simulink model "cube_2d_simulation_model_mpc"  (R2016b)
settings: Solver=VariableStepAuto  StartTime=0.0  StopTime=6  FixedStep=0.001  RelTol=1e-3  EnableMultiTasking=on
PreLoadFcn:
  | cubeinit
InitFcn:
  | cubeparameters
values from neighbouring files (symbols this model uses):
  g = 9.81    [MPC_Parameters.m]
  x0 = [deg2rad(2) 0]'    [MPC_init.m]    (also in MPC_simulation_linearized_system.m; MPC_simulation_nonlinearized_system.m; fastMPC.m)
undefined symbols (not defined in the file or in its folder): a_max, a_scaling, cube, deg_, imu_intended_alignment, imu_misalignment, motor, r_cube2imu, sensor_seed, T_onboard, Ts, w_max, w_scaling, wheel
libraries: cube_lib x9, simulink x6, cubex_simulation x3, stm32f4_io_lib x2
settings Model: Creator=Stefan  LastModifiedBy=Wall
settings DataIOCC: LimitDataPoints=on
settings OptimizationCC: LifeSpan=inf
settings DebuggingCC: AlgebraicLoopMsg=none  AllowSymbolicDim=off  SFUnexpectedBacktrackingDiag=warning  SFNoUnconditionalDefaultTransitionDiag=warning  SFExecutionAtInitializationDiag=none
settings ModelReferenceCC: PropagateSignalLabelsOutOfModel=off
settings GRTTargetCC: TargetLangStandard=C89/C90 (ANSI)
settings ConfigComp: CovMetricSettings=dw  CovHtmlReporting=on  CovSaveCumulativeToWorkspaceVar=on  CovSaveSingleToWorkspaceVar=on  CovExternalEMLEnable=off

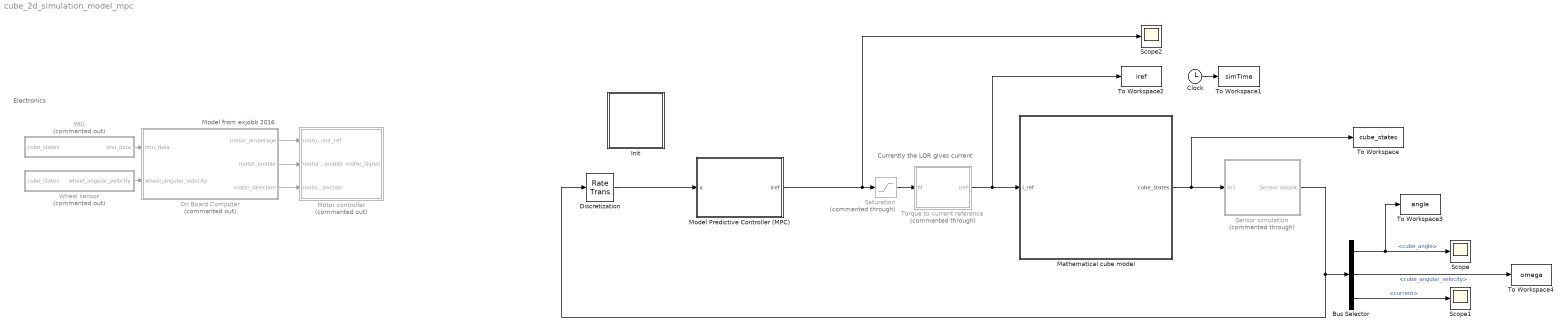
== system cube_2d_simulation_model_mpc ==
  note: Currently the LQR gives current
  note: Model from exjobb 2016
  note: Electronics
  Bus Selector : BusSelector  OutputSignals=cube_angle,cube_angular_velocity,motorStates.current
  Clock : Clock
  "Discretization " : RateTransition  OutPortSampleTime=Ts.controller
  IMU : Subsystem  Commented=on
  Init : Subsystem  InitFcn=cubeinit
  Mathematical cube model : Subsystem
      settings: MinAlgLoopOccurrences=on
  Model Predictive Controller (MPC) : Subsystem
  Motor controller : Subsystem  Commented=on
  On Board Computer : Subsystem  Commented=on
  Saturation : Saturate  Commented=through  UpperLimit=motor.Imax  LowerLimit=-motor.Imax
  Scope : Scope
  Scope1 : Scope
  Scope2 : Scope
  Sensor simulation : Subsystem  Commented=through
  To Workspace : ToWorkspace  VariableName=cube_states  SaveFormat=Timeseries  SampleTime=-1
  To Workspace1 : ToWorkspace  VariableName=simTime  SaveFormat=Timeseries  SampleTime=-1
  To Workspace2 : ToWorkspace  VariableName=iref  SaveFormat=Timeseries  SampleTime=-1
  To Workspace3 : ToWorkspace  VariableName=angle  SaveFormat=Timeseries  SampleTime=-1
  To Workspace4 : ToWorkspace  VariableName=omega  SaveFormat=Timeseries  SampleTime=-1
  Torque to current reference : Subsystem  Commented=through
  Wheel sensor : Subsystem  Commented=on
  wires:
  Mathematical cube model/1(cube_states) -> To Workspace/1, Sensor simulation/1(In1)
  On Board Computer/3(motor_direction) -> Motor controller/3(motor_direction)
  On Board Computer/1(motor_amperage) -> Motor controller/1(motor_current_ref)
  On Board Computer/2(motor_enable) -> Motor controller/2(motor_enable)
  Wheel sensor/1(wheel_angular_velocity) -> On Board Computer/2(wheel_angular_velocity)
  IMU/1(imu_data) -> On Board Computer/1(imu_data)
  "Discretization "/1 -> Model Predictive Controller (MPC)/1(x)
  Clock/1 -> To Workspace1/1
  Saturation/1 -> Torque to current reference/1(M)
  Bus Selector/1 -> To Workspace3/1, Scope/1  "<cube_angle>"
  Bus Selector/3 -> Scope1/1  "<current>"
  Torque to current reference/1(iref) -> To Workspace2/1, Mathematical cube model/1(i_ref)
  Sensor simulation/1(Sensor output) -> "Discretization "/1, Bus Selector/1
  Bus Selector/2 -> To Workspace4/1  "<cube_angular_velocity>"
  Model Predictive Controller (MPC)/1(iref) -> Scope2/1, Saturation/1

== system cube_2d_simulation_model_mpc/IMU ==
  cube_states : Inport
  Add IMU errors : Subsystem
  Convert to IMU output : Subsystem
  To Workspace : ToWorkspace  VariableName=imu_data  SaveFormat=Timeseries  SampleTime=-1
  Transform cube states to IMU states (adds gravity) : MATLAB Function  TreatAsAtomicUnit=on
  imu_data : Outport
  wires:
  cube_states/1 -> Transform cube states to IMU states (adds gravity)/1(cube_states)
  Transform cube states to IMU states (adds gravity)/1(imu_states) -> Add IMU errors/1(true_states)
  Add IMU errors/1(measured_states) -> Convert to IMU output/1(measured_output)
  Convert to IMU output/1(imu_output) -> To Workspace/1, imu_data/1

== system cube_2d_simulation_model_mpc/Init ==
  Constant3 : Constant
  Terminator : Terminator
  wires:
  Constant3/1 -> Terminator/1

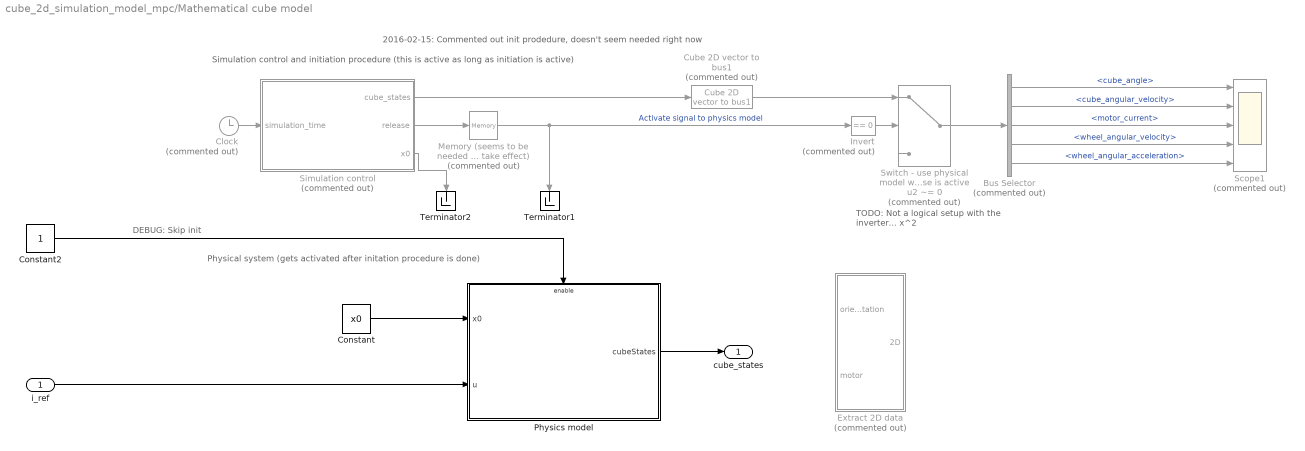
== system cube_2d_simulation_model_mpc/Mathematical cube model ==
  note: DEBUG: Skip init
  note: 2016-02-15: Commented out init prodedure, doesn't seem needed right now
  note: TODO: Not a logical setup
      | with the inverter... x^2
  note: Simulation control and initiation procedure (this is active as long as initiation is active)
  note: Physical system (gets activated after initation procedure is done)
  i_ref : Inport
  Bus Selector : BusSelector  Commented=on  OutputSignals=cube_angle,cube_angular_velocity,motor_current,wheel_angular_velocity,wheel_angular_acceleration
  Clock : Clock  Commented=on
  Constant : Constant  Value=x0  VectorParams1D=off
  Constant2 : Constant
  Cube 2D vector to bus1 : cube_lib/Cube 2D vector to bus1  Commented=on
  Extract 2D data : Subsystem  Commented=on
  Invert : simulink/Logic and Bit Operations/Compare To Constant  Commented=on  relop===  const=0  OutDataTypeStr=boolean
  Memory (seems to be needed for x0 to take effect) : Memory  Commented=on
  Physics model : Subsystem  TreatAsAtomicUnit=on
  Scope1 : Scope  Commented=on  NumInputPorts=5
  Simulation control : MATLAB Function  Commented=on  TreatAsAtomicUnit=on
  Switch - use physical model when release is active : Switch  Commented=on  Criteria=u2 ~= 0
  Terminator1 : Terminator
  Terminator2 : Terminator
  cube_states : Outport
  wires:
  Bus Selector/2 -> Scope1/2  "<cube_angular_velocity>"
  Bus Selector/1 -> Scope1/1  "<cube_angle>"
  Bus Selector/4 -> Scope1/4  "<wheel_angular_velocity>"
  Bus Selector/5 -> Scope1/5  "<wheel_angular_acceleration>"
  Bus Selector/3 -> Scope1/3  "<motor_current>"
  Clock/1 -> Simulation control/1(simulation_time)
  Simulation control/2(release) -> Memory (seems to be needed for x0 to take effect)/1
  Simulation control/1(cube_states) -> Cube 2D vector to bus1/1
  Cube 2D vector to bus1/1 -> Switch - use physical model when release is active/1
  Switch - use physical model when release is active/1 -> Bus Selector/1
  Simulation control/3(x0) -> Terminator2/1
  Invert/1 -> Switch - use physical model when release is active/2
  Memory (seems to be needed for x0 to take effect)/1 -> Invert/1, Terminator1/1  "Activate signal to physics model"
  i_ref/1 -> Physics model/2(u)
  Constant2/1 -> Physics model/Enable
  Physics model/1("cubeStates ") -> cube_states/1
  Constant/1 -> Physics model/1("x0 ")

== system cube_2d_simulation_model_mpc/Model Predictive Controller (MPC) ==
  x : Inport
  Bus Selector2 : BusSelector  OutputSignals=cube_angle,cube_angular_velocity
  MPC : MATLAB Function  TreatAsAtomicUnit=on
  iref : Outport
  wires:
  Bus Selector2/2 -> MPC/2(cube_angular_velocity)  "<cube_angular_velocity>"
  x/1 -> Bus Selector2/1
  Bus Selector2/1 -> MPC/1(cube_angle)  "<cube_angle>"
  MPC/1(iref) -> iref/1

== system cube_2d_simulation_model_mpc/Motor controller ==
  note: Basically, the onboard computer does exactly this but inverted.
      | The conversion and inversion are done to be able to simulate real onboard computer behaviour.
  note: Convert direction to -1/1
  note: 0 (backward) / 1 (forward)
  note: 0/1
  note: Absolute value
  motor_current_ref : Inport
  motor_enable : Inport  Port=2
  motor_direction : Inport  Port=3
  Add : Sum
  Constant : Constant  Value=-1
  Gain : Gain  Gain=2
  Product : Product  Inputs=3
  motor_signal : Outport
  wires:
  motor_enable/1 -> Product/2
  motor_current_ref/1 -> Product/1
  Product/1 -> motor_signal/1
  Constant/1 -> Add/1
  motor_direction/1 -> Gain/1
  Gain/1 -> Add/2
  Add/1 -> Product/3

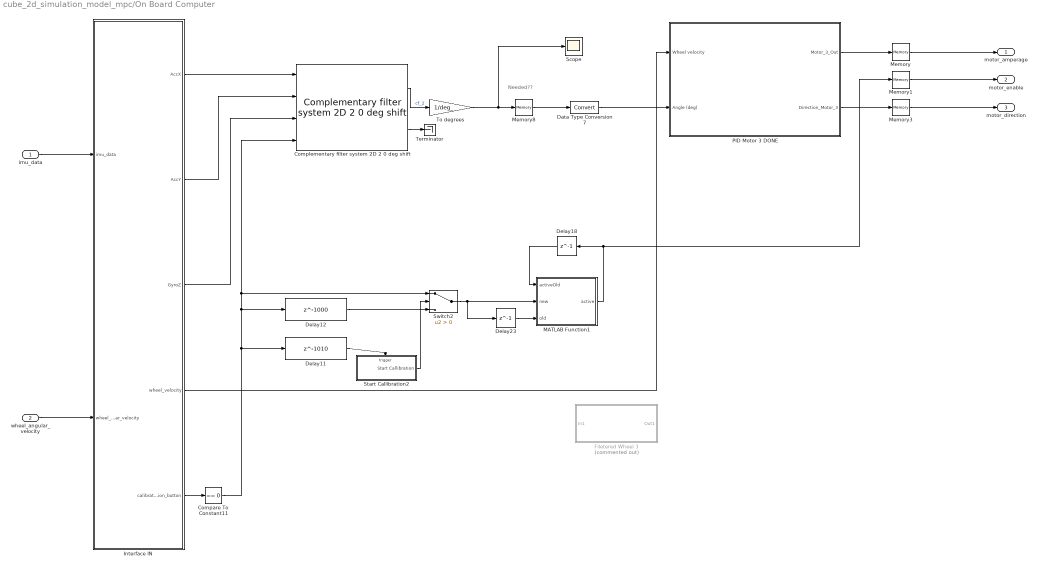
== system cube_2d_simulation_model_mpc/On Board Computer ==
  note: Needed??
  imu_data : Inport
  wheel_angular_velocity : Inport  Port=2
  Compare To Constant11 : simulink/Logic and Bit Operations/Compare To Constant  relop===  const=0  OutDataTypeStr=boolean  ZeroCross=off
  Complementary filter system 2D 2 0 deg shift : cube_lib/Complementary filter system 2D 2 0 deg shift
  Data Type Conversion7 : DataTypeConversion
  Delay11 : Delay  DelayLength=1010  InitialCondition=0
  Delay12 : Delay  DelayLength=1000  InitialCondition=0
  Delay18 : Delay  DelayLength=1  InitialCondition=0
  Delay23 : Delay  DelayLength=1  InitialCondition=0
  Filetered Wheel 3 : Subsystem  Commented=on
  Interface IN : Subsystem
  MATLAB Function1 : MATLAB Function  TreatAsAtomicUnit=on
  Memory{,1,3,8} (4 alike) : Memory  InheritSampleTime=on
  "PID Motor 3 DONE " : Subsystem
  Scope : Scope
  Start Callibration2 : Subsystem
  Switch2 : Switch  Criteria=u2 > Threshold
  Terminator : Terminator
  To degrees : Gain  Gain=1/deg_
  motor_amperage : Outport
  motor_enable : Outport  Port=2
  motor_direction : Outport  Port=3
  wires:
  imu_data/1 -> Interface IN/1(imu_data)
  Data Type Conversion7/1 -> "PID Motor 3 DONE "/2(Angle (deg))
  "PID Motor 3 DONE "/1(Motor_3_Out) -> Memory/1
  Memory8/1 -> Data Type Conversion7/1
  "PID Motor 3 DONE "/2("Direction_Motor_3 ") -> Memory3/1
  Compare To Constant11/1 -> Delay12/1, Complementary filter system 2D 2 0 deg shift/4, Switch2/1, Delay11/1
  MATLAB Function1/1(active) -> Memory1/1, Delay18/1
  Delay23/1 -> MATLAB Function1/3(old)
  Switch2/1 -> Delay23/1, MATLAB Function1/2(new)
  Delay18/1 -> MATLAB Function1/1(activeOld)
  Start Callibration2/1(Start Callibration) -> Switch2/2
  Delay11/1 -> Start Callibration2/Trigger
  Delay12/1 -> Switch2/3
  wheel_angular_velocity/1 -> Interface IN/2(wheel_angular_velocity)
  Memory/1 -> motor_amperage/1
  Memory1/1 -> motor_enable/1
  Memory3/1 -> motor_direction/1
  Interface IN/5(calibration_button) -> Compare To Constant11/1
  Interface IN/4(wheel_velocity) -> "PID Motor 3 DONE "/1(Wheel velocity)
  Interface IN/1(AccX) -> Complementary filter system 2D 2 0 deg shift/1
  Interface IN/2("AccY ") -> Complementary filter system 2D 2 0 deg shift/2
  Interface IN/3(GyroZ) -> Complementary filter system 2D 2 0 deg shift/3
  Complementary filter system 2D 2 0 deg shift/1 -> To degrees/1  "cf_2"
  To degrees/1 -> Scope/1, Memory8/1
  Complementary filter system 2D 2 0 deg shift/2 -> Terminator/1

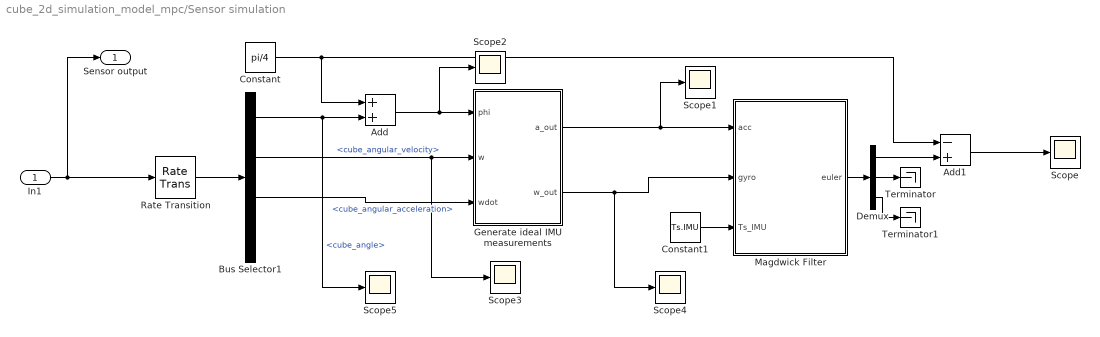
== system cube_2d_simulation_model_mpc/Sensor simulation ==
  In1 : Inport
  Add : Sum
  Add1 : Sum  Inputs=-+
  Bus Selector1 : BusSelector  OutputSignals=cube_angle,cube_angular_velocity,cube_angular_acceleration,motorStates
  Constant : Constant  Value=pi/4
  Constant1 : Constant  Value=Ts.IMU
  Demux : Demux  Outputs=3
  Generate ideal IMU measurements : MATLAB Function  TreatAsAtomicUnit=on
  Magdwick Filter : MATLAB Function  TreatAsAtomicUnit=on
  Rate Transition : RateTransition  OutPortSampleTime=Ts.IMU
  Scope{,1..5} (6 alike) : Scope
  Terminator : Terminator
  Terminator1 : Terminator
  Sensor output : Outport
  wires:
  In1/1 -> Rate Transition/1, Sensor output/1
  Bus Selector1/1 -> Scope5/1, Add/2  "<cube_angle>"
  Bus Selector1/2 -> Scope3/1, Generate ideal IMU measurements/2(w)  "<cube_angular_velocity>"
  Bus Selector1/3 -> Generate ideal IMU measurements/3(wdot)  "<cube_angular_acceleration>"
  Constant/1 -> Add1/1, Add/1
  Add/1 -> Scope2/1, Generate ideal IMU measurements/1(phi)
  Constant1/1 -> Magdwick Filter/3(Ts_IMU)
  Generate ideal IMU measurements/1(a_out) -> Scope1/1, Magdwick Filter/1(acc)
  Generate ideal IMU measurements/2(w_out) -> Scope4/1, Magdwick Filter/2(gyro)
  Magdwick Filter/1(euler) -> Demux/1
  Demux/1 -> Add1/2
  Add1/1 -> Scope/1
  Demux/2 -> Terminator/1
  Demux/3 -> Terminator1/1
  Rate Transition/1 -> Bus Selector1/1

== system cube_2d_simulation_model_mpc/Torque to current reference ==
  note: The LQR synthesis is designed so that the controller outputs a moment in newton-meters.
      | For the real system this should be a conversion function from moment to the PWM signal used by the Maxxon ESC.
  M : Inport
  Moment to current : Gain  Gain=1/motor.kt
  iref : Outport
  wires:
  Moment to current/1 -> iref/1
  M/1 -> Moment to current/1

== system cube_2d_simulation_model_mpc/Wheel sensor ==
  cube_states : Inport
  Bus Selector : BusSelector  OutputSignals=wheel_angular_velocity
  Sensor : cube_lib/Sensor  scale_factor=1  bias=0  noise_std=wheel_noise_standard_deviation  noise_seed=wheel_sensor_seed  sample_time=T_onboard
  wheel_angular_velocity : Outport
  wires:
  Sensor/1 -> wheel_angular_velocity/1
  cube_states/1 -> Bus Selector/1
  Bus Selector/1 -> Sensor/1  "<wheel_angular_velocity>"

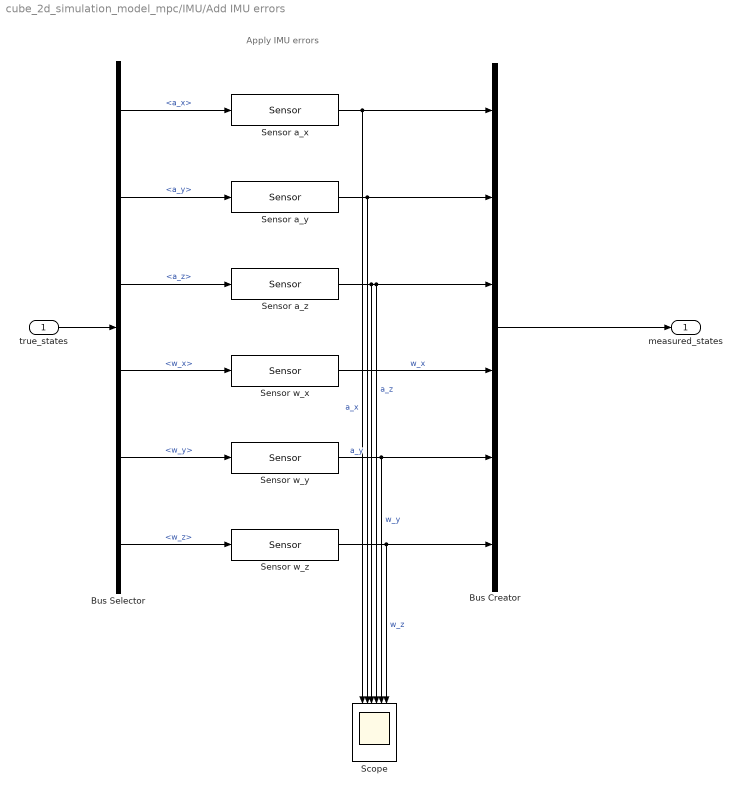
== system cube_2d_simulation_model_mpc/IMU/Add IMU errors ==
  note: Apply IMU errors
  true_states : Inport
  Bus Creator : BusCreator  Inputs=6  OutDataTypeStr=Bus: ImuStates
  Bus Selector : BusSelector  OutputSignals=a_x,a_y,a_z,w_x,w_y,w_z
  Scope : Scope  NumInputPorts=6
  Sensor a_x : cube_lib/Sensor  scale_factor=imu_scale_factor_a_x  bias=imu_bias_a_x  noise_std=imu_noise_a_standard_deviation  noise_seed=sensor_seed  sample_time=T_onboard
  Sensor a_y : cube_lib/Sensor  scale_factor=imu_scale_factor_a_y  bias=imu_bias_a_y  noise_std=imu_noise_a_standard_deviation  noise_seed=sensor_seed+1  sample_time=T_onboard
  Sensor a_z : cube_lib/Sensor  scale_factor=imu_scale_factor_a_z  bias=imu_bias_a_z  noise_std=imu_noise_a_standard_deviation  noise_seed=sensor_seed+2  sample_time=T_onboard
  Sensor w_x : cube_lib/Sensor  scale_factor=imu_scale_factor_w_x  bias=imu_bias_w_x  noise_std=imu_noise_w_standard_deviation  noise_seed=sensor_seed+3  sample_time=T_onboard
  Sensor w_y : cube_lib/Sensor  scale_factor=imu_scale_factor_w_y  bias=imu_bias_w_y  noise_std=imu_noise_w_standard_deviation  noise_seed=sensor_seed+4  sample_time=T_onboard
  Sensor w_z : cube_lib/Sensor  scale_factor=imu_scale_factor_w_z  bias=imu_bias_w_z  noise_std=imu_noise_w_standard_deviation  noise_seed=sensor_seed+5  sample_time=T_onboard
  measured_states : Outport
  wires:
  Bus Creator/1 -> measured_states/1
  true_states/1 -> Bus Selector/1
  Bus Selector/6 -> Sensor w_z/1  "<w_z>"
  Sensor a_x/1 -> Scope/1, Bus Creator/1  "a_x"
  Bus Selector/2 -> Sensor a_y/1  "<a_y>"
  Bus Selector/4 -> Sensor w_x/1  "<w_x>"
  Sensor a_y/1 -> Bus Creator/2, Scope/2  "a_y"
  Sensor w_x/1 -> Bus Creator/4  "w_x"
  Sensor w_y/1 -> Bus Creator/5, Scope/5  "w_y"
  Sensor w_z/1 -> Bus Creator/6, Scope/6  "w_z"
  Sensor a_z/1 -> Bus Creator/3, Scope/4, Scope/3  "a_z"
  Bus Selector/5 -> Sensor w_y/1  "<w_y>"
  Bus Selector/3 -> Sensor a_z/1  "<a_z>"
  Bus Selector/1 -> Sensor a_x/1  "<a_x>"

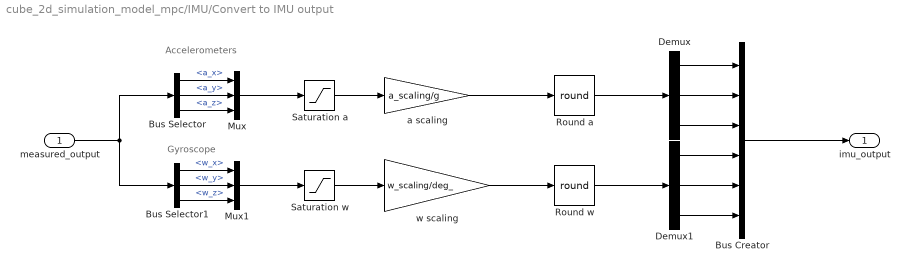
== system cube_2d_simulation_model_mpc/IMU/Convert to IMU output ==
  note: Gyroscope
  note: Accelerometers
  measured_output : Inport
  Bus Creator : BusCreator  Inputs=6  OutDataTypeStr=Bus: ImuStates
      settings: InheritFromInputs=off
  Bus Selector : BusSelector  OutputSignals=a_x,a_y,a_z
  Bus Selector1 : BusSelector  OutputSignals=w_x,w_y,w_z
  Demux : Demux  Outputs=3
  Demux1 : Demux  Outputs=3
  Mux : Mux  Inputs=3
  Mux1 : Mux  Inputs=3
  Round a : Rounding  Operator=round
  Round w : Rounding  Operator=round
  Saturation a : Saturate  UpperLimit=a_max  LowerLimit=-a_max
  Saturation w : Saturate  UpperLimit=w_max  LowerLimit=-w_max
  a scaling : Gain  Gain=a_scaling/g
  w scaling : Gain  Gain=w_scaling/deg_
  imu_output : Outport
  wires:
  measured_output/1 -> Bus Selector1/1, Bus Selector/1
  a scaling/1 -> Round a/1
  Saturation a/1 -> a scaling/1
  Saturation w/1 -> w scaling/1
  w scaling/1 -> Round w/1
  Bus Creator/1 -> imu_output/1
  Bus Selector/2 -> Mux/2  "<a_y>"
  Bus Selector/3 -> Mux/3  "<a_z>"
  Bus Selector/1 -> Mux/1  "<a_x>"
  Mux/1 -> Saturation a/1
  Bus Selector1/2 -> Mux1/2  "<w_y>"
  Bus Selector1/3 -> Mux1/3  "<w_z>"
  Bus Selector1/1 -> Mux1/1  "<w_x>"
  Mux1/1 -> Saturation w/1
  Round a/1 -> Demux/1
  Round w/1 -> Demux1/1
  Demux/3 -> Bus Creator/3
  Demux/1 -> Bus Creator/1
  Demux/2 -> Bus Creator/2
  Demux1/3 -> Bus Creator/6
  Demux1/2 -> Bus Creator/5
  Demux1/1 -> Bus Creator/4

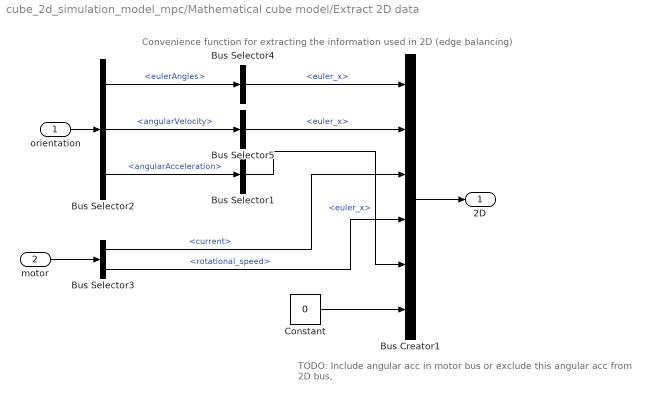
== system cube_2d_simulation_model_mpc/Mathematical cube model/Extract 2D data ==
  note: TODO: Include angular acc in motor bus or exclude this angular acc
      | 	     from 2D bus,
  note: Convenience function for extracting the information used in 2D (edge balancing)
  orientation : Inport  OutDataTypeStr=Bus: orientation
  motor : Inport  Port=2
  Bus Creator1 : BusCreator  Inputs=6  OutDataTypeStr=Bus: CubeStates2D
      settings: InheritFromInputs=off
  Bus Selector1 : BusSelector  OutputSignals=euler_x
  Bus Selector2 : BusSelector  OutputSignals=eulerAngles,angularVelocity,angularAcceleration
  Bus Selector3 : BusSelector  OutputSignals=current,rotational_speed
  Bus Selector4 : BusSelector  OutputSignals=euler_x
  Bus Selector5 : BusSelector  OutputSignals=euler_x
  Constant : Constant  Value=0
  2D : Outport  OutDataTypeStr=Bus: CubeStates2D
  wires:
  Bus Selector2/2 -> Bus Selector5/1  "<angularVelocity>"
  Bus Selector3/1 -> Bus Creator1/3  "<current>"
  Bus Selector4/1 -> Bus Creator1/1  "<euler_x>"
  Bus Selector5/1 -> Bus Creator1/2  "<euler_x>"
  Bus Creator1/1 -> 2D/1
  Bus Selector2/1 -> Bus Selector4/1  "<eulerAngles>"
  orientation/1 -> Bus Selector2/1
  Bus Selector3/2 -> Bus Creator1/4  "<rotational_speed>"
  motor/1 -> Bus Selector3/1
  Bus Selector2/3 -> Bus Selector1/1  "<angularAcceleration>"
  Bus Selector1/1 -> Bus Creator1/5  "<euler_x>"
  Constant/1 -> Bus Creator1/6

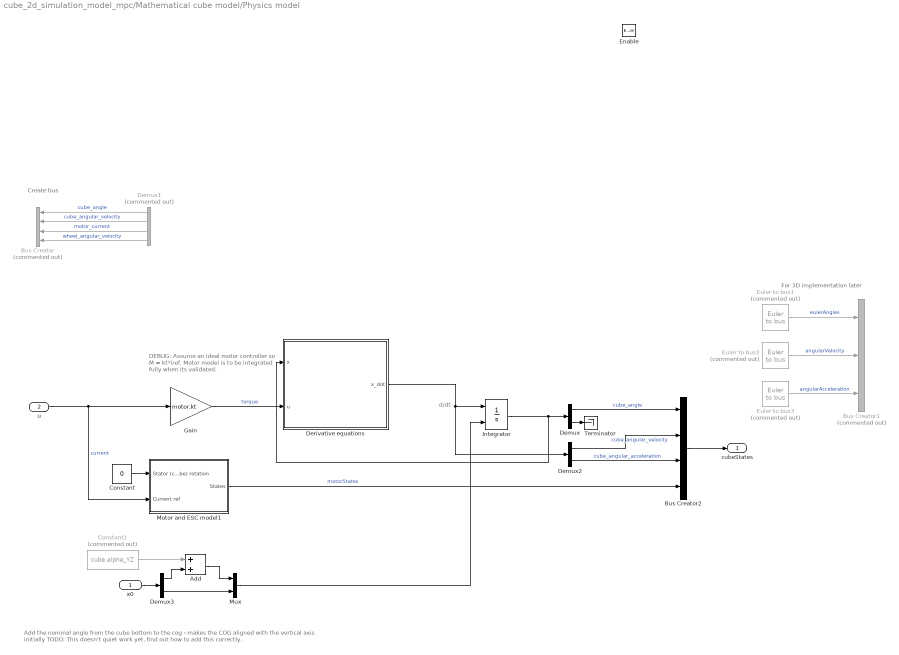
== system cube_2d_simulation_model_mpc/Mathematical cube model/Physics model ==
  note: Add the nominal angle from the cube bottom to the cog - makes the COG aligned with the vertical axis initially
      | TODO: This doesn't quiet work yet, find out how to add this correctly.
  note: DEBUG: Assume an ideal motor
      | controller so M = kt*iref. Motor model
      | is to be integrated fully when its validated.
  note: For 3D implementation later
  note: d/dt
  note: Create bus
  "x0 " : Inport
  u : Inport  Port=2
  Enable : EnablePort
  Add : Sum
  Bus Creator1 : BusCreator  Commented=on  Inputs='eulerAngles','angularVelocity','angularAcceleration'  OutDataTypeStr=Bus: orientation
  Bus Creator2 : BusCreator  Inputs='cube_angle','cube_angular_velocity','cube_angular_acceleration','motorStates'  OutDataTypeStr=Bus: CubeStates2D
  Bus Creator : BusCreator  Commented=on  Inputs=4  OutDataTypeStr=Bus: statevector
  Constant : Constant  Value=0
  Constant1 : Constant  Commented=on  Value=cube.alpha_YZ
  Demux : Demux  Outputs=2
  Demux1 : Demux  Commented=on
  Demux2 : Demux  Outputs=2
  Demux3 : Demux  Outputs=2
  Derivative equations : MATLAB Function
  Euler to bus1 : cubex_simulation/Euler to bus  Commented=on
  Euler to bus2 : cubex_simulation/Euler to bus  Commented=on
  Euler to bus3 : cubex_simulation/Euler to bus  Commented=on
  Gain : Gain  Gain=motor.kt
  Integrator : Integrator  InitialConditionSource=external
  Motor and ESC model1 : Subsystem  AncestorBlock=cubex_simulation/Motor and ESC model
  Mux : Mux  Inputs=2
  Terminator : Terminator
  "cubeStates " : Outport
  wires:
  Demux1/1 -> Bus Creator/1  "cube_angle"
  Demux1/2 -> Bus Creator/2  "cube_angular_velocity"
  Demux1/4 -> Bus Creator/4  "wheel_angular_velocity"
  Demux1/3 -> Bus Creator/3  "motor_current"
  Integrator/1 -> Demux/1, Derivative equations/1(x)
  Derivative equations/1(x_dot) -> Demux2/1, Integrator/1
  Euler to bus1/1 -> Bus Creator1/1  "eulerAngles"
  Euler to bus2/1 -> Bus Creator1/2  "angularVelocity"
  Euler to bus3/1 -> Bus Creator1/3  "angularAcceleration"
  Demux/1 -> Bus Creator2/1  "cube_angle"
  Bus Creator2/1 -> "cubeStates "/1
  Demux2/1 -> Bus Creator2/2  "cube_angular_velocity"
  Demux2/2 -> Bus Creator2/3  "cube_angular_acceleration"
  Demux/2 -> Terminator/1
  u/1 -> Motor and ESC model1/2(Current ref), Gain/1  "current"
  Motor and ESC model1/1("States ") -> Bus Creator2/4  "motorStates"
  Gain/1 -> Derivative equations/2(u)  "torque"
  Constant/1 -> Motor and ESC model1/1(Stator (cube) rotation)
  "x0 "/1 -> Demux3/1
  Add/1 -> Mux/1
  Demux3/2 -> Mux/2
  Demux3/1 -> Add/2
  Constant1/1 -> Add/1
  Mux/1 -> Integrator/2

== system cube_2d_simulation_model_mpc/On Board Computer/Filetered Wheel 3 ==
  In1 : Inport
  Add3 : Sum  Inputs=-+
  Add9 : Sum  Inputs=-+
  Constant1 : Constant  Value=2094  SampleTime=-1
  Constant15 : Constant  Value=69  SampleTime=-1
  Gain2 : Gain  Gain=(6110*2)/4096
  RPM to RAD3 : Gain  Gain=1/9.55
  Scope : Scope
  Out1 : Outport
  wires:
  Gain2/1 -> RPM to RAD3/1
  Add3/1 -> Gain2/1
  Constant1/1 -> Add3/1
  In1/1 -> Add3/2
  Constant15/1 -> Add9/1
  RPM to RAD3/1 -> Add9/2
  Add9/1 -> Scope/1, Out1/1

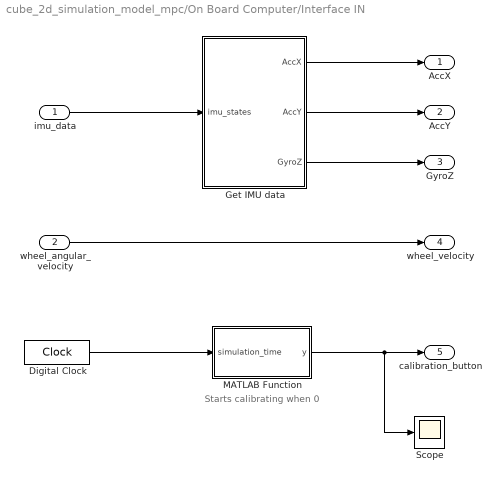
== system cube_2d_simulation_model_mpc/On Board Computer/Interface IN ==
  note: Starts calibrating when 0
  imu_data : Inport
  wheel_angular_velocity : Inport  Port=2
  Digital Clock : DigitalClock  SampleTime=T_onboard
  Get IMU data : Subsystem
  MATLAB Function : MATLAB Function  TreatAsAtomicUnit=on
  Scope : Scope
  AccX : Outport
  "AccY " : Outport  Port=2
  GyroZ : Outport  Port=3
  wheel_velocity : Outport  Port=4
  calibration_button : Outport  Port=5
  wires:
  wheel_angular_velocity/1 -> wheel_velocity/1
  imu_data/1 -> Get IMU data/1(imu_states)
  Get IMU data/1(AccX) -> AccX/1
  Get IMU data/2("AccY ") -> "AccY "/1
  Get IMU data/3(GyroZ) -> GyroZ/1
  MATLAB Function/1(y) -> Scope/1, calibration_button/1
  Digital Clock/1 -> MATLAB Function/1(simulation_time)

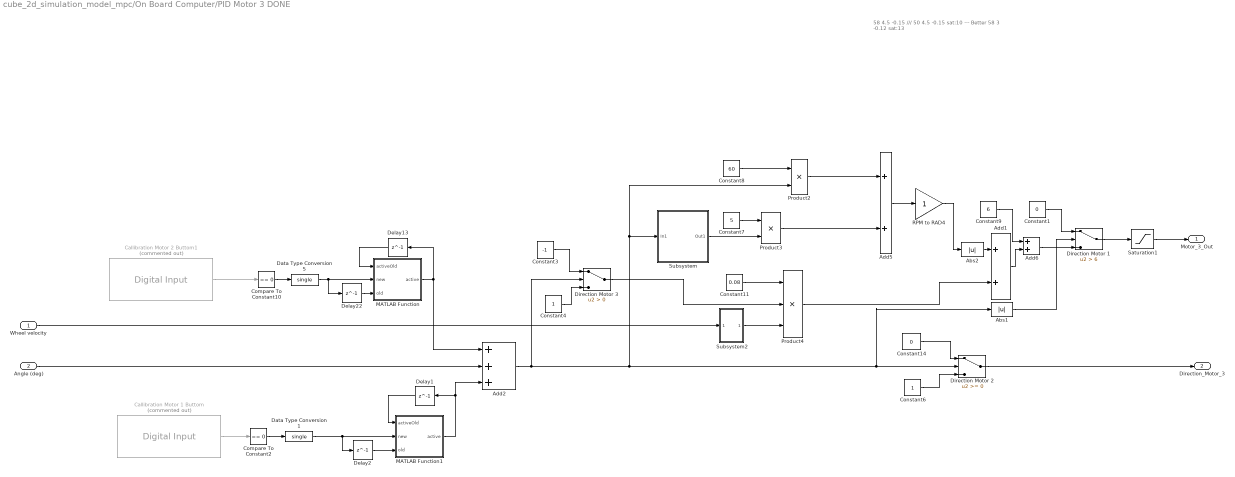
== system cube_2d_simulation_model_mpc/On Board Computer/PID Motor 3 DONE  ==
  note: 58
      | 4.5
      | -0.15
      | ///
      | 50
      | 4.5
      | -0.15
      | sat:10
      | --- Better
      | 58
      | 3
      | -0.12
      | sat:13
  Wheel velocity : Inport
  Angle (deg) : Inport  Port=2
  Abs1 : Abs
  Abs2 : Abs
  Add1 : Sum
  Add2 : Sum  Inputs=+++
  Add5 : Sum
  Add6 : Sum
  Callibration Motor 1 Buttom : stm32f4_io_lib/Digital Input  Commented=on  port=E  speed=100  porttype=Pull Up  porttypestr=UP  use_pin0=off  use_pin1=off  use_pin2=off  use_pin3=off  use_pin4=off  use_pin5=off  use_pin6=off  use_pin7=off  use_pin8=off  use_pin9=off  use_pin10=off  use_pin11=off  use_pin12=off  use_pin13=off  use_pin14=on  use_pin15=off  pinstr=GPIO_Pin_14  usedpinarray="[0  0  0  0  0  0  0  0  0  0  0  0  0  0  1  0]"  bitbandingstr="#define OnBoardComputerPIDMotor3DONECallibrationMotor1Buttom_E14 Peripheral_BB(GPIOE->IDR, 14)  /* Output pin */"  sampletime=0.002  sampletimestr=0.002  blockid=OnBoardComputerPIDMotor3DONECallibrationMotor1Buttom  enablecustomportlabel=off  glabalinit=off  cinputportlabel=In1, In2  coutputportlabel=Out1, Out2
  Callibration Motor 2 Buttom1 : stm32f4_io_lib/Digital Input  Commented=on  port=E  speed=100  porttype=Pull Up  porttypestr=UP  use_pin0=off  use_pin1=off  use_pin2=off  use_pin3=off  use_pin4=off  use_pin5=off  use_pin6=off  use_pin7=off  use_pin8=off  use_pin9=off  use_pin10=off  use_pin11=on  use_pin12=off  use_pin13=off  use_pin14=off  use_pin15=off  pinstr=GPIO_Pin_11  usedpinarray="[0  0  0  0  0  0  0  0  0  0  0  1  0  0  0  0]"  bitbandingstr="#define OnBoardComputerPIDMotor3DONECallibrationMotor2Buttom1_E11 Peripheral_BB(GPIOE->IDR, 11)  /* Output pin */"  sampletime=0.002  sampletimestr=0.002  blockid=OnBoardComputerPIDMotor3DONECallibrationMotor2Buttom1  enablecustomportlabel=off  glabalinit=off  cinputportlabel=In1, In2  coutputportlabel=Out1, Out2
  Compare To Constant10 : simulink/Logic and Bit Operations/Compare To Constant  relop===  const=0  OutDataTypeStr=boolean  ZeroCross=off
  Compare To Constant2 : simulink/Logic and Bit Operations/Compare To Constant  relop===  const=0  OutDataTypeStr=boolean  ZeroCross=off
  Constant1 : Constant  Value=0  OutDataTypeStr=single  SampleTime=-1
  Constant11 : Constant  Value=0.08  OutDataTypeStr=single  SampleTime=-1
  Constant14 : Constant  Value=0  OutDataTypeStr=single  SampleTime=-1
  Constant3 : Constant  Value=-1  OutDataTypeStr=single  SampleTime=-1
  Constant4 : Constant  OutDataTypeStr=single  SampleTime=-1
  Constant6 : Constant  OutDataTypeStr=single  SampleTime=-1
  Constant7 : Constant  Value=5  OutDataTypeStr=single  SampleTime=-1
  Constant8 : Constant  Value=60  OutDataTypeStr=single  SampleTime=-1
  Constant9 : Constant  Value=6  SampleTime=-1
  Data Type Conversion1 : DataTypeConversion  OutDataTypeStr=single
  Data Type Conversion5 : DataTypeConversion  OutDataTypeStr=single
  Delay{1..2,13,22} (4 alike) : Delay  DelayLength=1  InitialCondition=0
  Direction Motor 1 : Switch  Criteria=u2 > Threshold  Threshold=6
  Direction Motor 2 : Switch
  Direction Motor 3 : Switch  Criteria=u2 > Threshold
  MATLAB Function : MATLAB Function  TreatAsAtomicUnit=on
  MATLAB Function1 : MATLAB Function  TreatAsAtomicUnit=on
  Product2 : Product
  Product3 : Product
  Product4 : Product  Inputs=3
  RPM to RAD4 : Gain
  Saturation1 : Saturate  UpperLimit=90  LowerLimit=10
  Subsystem : Subsystem
  Subsystem2 : Subsystem
  Motor_3_Out : Outport
  "Direction_Motor_3 " : Outport  Port=2
  wires:
  Direction Motor 2/1 -> "Direction_Motor_3 "/1
  Constant7/1 -> Product3/1
  Constant11/1 -> Product4/1
  Constant14/1 -> Direction Motor 2/1
  Constant6/1 -> Direction Motor 2/3
  Product3/1 -> Add5/2
  Constant9/1 -> Add6/1
  Add5/1 -> RPM to RAD4/1
  RPM to RAD4/1 -> Abs2/1
  Product2/1 -> Add5/1
  Abs2/1 -> Add1/1
  Saturation1/1 -> Motor_3_Out/1
  Constant8/1 -> Product2/1
  Add6/1 -> Direction Motor 1/3
  Direction Motor 1/1 -> Saturation1/1
  Constant1/1 -> Direction Motor 1/1
  Abs1/1 -> Direction Motor 1/2
  Product4/1 -> Add1/2
  Wheel velocity/1 -> Subsystem2/1(In1)
  Angle (deg)/1 -> Add2/2
  Subsystem/1(Out1) -> Product3/2
  Add1/1 -> Add6/2
  Constant4/1 -> Direction Motor 3/3
  Constant3/1 -> Direction Motor 3/1
  Add2/1 -> Direction Motor 3/2, Subsystem/1(In1), Product2/2, Abs1/1, Direction Motor 2/2
  Callibration Motor 2 Buttom1/1 -> Compare To Constant10/1
  Compare To Constant10/1 -> Data Type Conversion5/1
  Callibration Motor 1 Buttom/1 -> Compare To Constant2/1
  Compare To Constant2/1 -> Data Type Conversion1/1
  MATLAB Function/1(active) -> Add2/1, Delay13/1
  Delay22/1 -> MATLAB Function/3(old)
  Data Type Conversion5/1 -> MATLAB Function/2(new), Delay22/1
  Delay13/1 -> MATLAB Function/1(activeOld)
  MATLAB Function1/1(active) -> Add2/3, Delay1/1
  Delay2/1 -> MATLAB Function1/3(old)
  Data Type Conversion1/1 -> Delay2/1, MATLAB Function1/2(new)
  Delay1/1 -> MATLAB Function1/1(activeOld)
  Subsystem2/1(Out2) -> Product4/3
  Direction Motor 3/1 -> Product4/2

== system cube_2d_simulation_model_mpc/On Board Computer/Start Callibration2 ==
  Trigger : TriggerPort  VariantControl=Variant  PortDimensions=1
  Constant2 : Constant
  Start Callibration : Outport  InitialOutput=[0]
  wires:
  Constant2/1 -> Start Callibration/1

== system cube_2d_simulation_model_mpc/Mathematical cube model/Physics model/Motor and ESC model1 ==
  note: The internal current loop is assumed faster then the rest of the system, and has another sampling rate therefore
  note: The Escon 36/3 motor controller contains an internal current PI controller in the operating mode used here.
  Stator (cube) rotation : Inport
  Current ref : Inport  Port=2
  Bus Creator : BusCreator  Inputs='current','torque','rotational_speed'  OutDataTypeStr=Bus: motorStates
  Discrete PID Controller : simulink/Continuous/PID Controller  Controller=PID  TimeDomain=Discrete-time  SampleTime=0.001  IntegratorMethod=Forward Euler  FilterMethod=Forward Euler  Form=Parallel  UseFilter=on  ControllerParametersSource=internal  P=3.61560541934839  I=475.697383940424  D=0.000607320932209109  N=593.755510731283  InitialConditionSource=internal  InitialConditionForIntegrator=0  InitialConditionForFilter=0  ExternalReset=none  LimitOutput=on  UpperSaturationLimit=motor.Vbat  LowerSaturationLimit=-motor.Vbat  LinearizeAsGain=on  AntiWindupMode=clamping  Kb=1  TrackingMode=off  Kt=1  PParamMin=[]  PParamMax=[]  IParamMin=[]  IParamMax=[]  DParamMin=[]  DParamMax=[]  NParamMin=[]  NParamMax=[]  KbParamMin=[]  KbParamMax=[]  KtParamMin=[]  KtParamMax=[]  POutMin=[]  POutMax=[]  IOutMin=[]  IOutMax=[]  DOutMin=[]  DOutMax=[]  NOutMin=[]  NOutMax=[]  KbOutMin=[]  KbOutMax=[]  KtOutMin=[]  KtOutMax=[]  IntegratorOutMin=[]  IntegratorOutMax=[]  FilterOutMin=[]  FilterOutMax=[]  SumOutMin=[]  SumOutMax=[]  SumI1OutMin=[]  SumI1OutMax=[]  SumI2OutMin=[]  SumI2OutMax=[]  SumI3OutMin=[]  SumI3OutMax=[]  SumDOutMin=[]  SumDOutMax=[]  SaturationOutMin=[]  SaturationOutMax=[]  IntegratorContinuousStateAttributes=''  IntegratorStateMustResolveToSignalObject=off  IntegratorRTWStateStorageClass=Auto  FilterContinuousStateAttributes=''  FilterStateMustResolveToSignalObject=off  FilterRTWStateStorageClass=Auto  DifferentiatorICPrevScaledInput=0  DifferentiatorOutMin=[]  DifferentiatorOutMax=[]
  Motor model : Subsystem
  Rate Transition : RateTransition  OutPortSampleTime=0.001
  Sum : Sum  Inputs=|+-
  Torque constant : Gain  Gain=motor.kt
  "States " : Outport  OutDataTypeStr=Bus: motorStates
  wires:
  Bus Creator/1 -> "States "/1
  Motor model/2(flywheel rotational speed) -> Bus Creator/3  "rotational_speed"
  Stator (cube) rotation/1 -> Motor model/2(Cube rotaion speed)
  Current ref/1 -> Rate Transition/1
  Discrete PID Controller/1 -> Motor model/1(Vin)
  Rate Transition/1 -> Sum/1
  Sum/1 -> Discrete PID Controller/1
  Torque constant/1 -> Bus Creator/2  "torque"
  Motor model/1(current) -> Bus Creator/1, Torque constant/1, Sum/2  "current"

== system cube_2d_simulation_model_mpc/On Board Computer/Interface IN/Get IMU data ==
  imu_states : Inport
  Bus Selector : BusSelector  OutputSignals=a_x,a_y,w_z
  AccX : Outport
  "AccY " : Outport  Port=2
  GyroZ : Outport  Port=3
  wires:
  imu_states/1 -> Bus Selector/1
  Bus Selector/1 -> AccX/1  "<a_x>"
  Bus Selector/2 -> "AccY "/1  "<a_y>"
  Bus Selector/3 -> GyroZ/1  "<w_z>"

== system cube_2d_simulation_model_mpc/On Board Computer/PID Motor 3 DONE /Subsystem ==
  In1 : Inport
  DUMMY7 : Terminator
  Discrete Derivative : simulink/Discrete/Discrete Derivative  gainval=1.0  ICPrevScaledInput=0.0  InputProcessing=Inherited  OutMin=[]  OutMax=[]  OutDataType=fixdt(1, 16)  OutScaling=2^-10  DoSatur=off
  Do average zero2 : If  NumInputs=2  IfExpression=u1 == u2
  Subsystem2 : Subsystem
  Unit Delay1 : UnitDelay  SampleTime=-1
  Out1 : Outport
  wires:
  Do average zero2/2 -> Subsystem2/Action
  Unit Delay1/1 -> Do average zero2/2
  Discrete Derivative/1 -> Out1/1  "Cube angle velocity [degree/s]"
  Subsystem2/1(Out1) -> Discrete Derivative/1
  In1/1 -> Subsystem2/1(In1), Unit Delay1/1, Do average zero2/1
  Do average zero2/1 -> DUMMY7/1

== system cube_2d_simulation_model_mpc/On Board Computer/PID Motor 3 DONE /Subsystem2 ==
  In1 : Inport
  DUMMY7 : Terminator
  Do average zero1 : If  NumInputs=2  IfExpression=u1 == u2
  Subsystem1 : Subsystem
  Unit Delay3 : UnitDelay  SampleTime=-1
  Out2 : Outport
  wires:
  Unit Delay3/1 -> Do average zero1/2
  Do average zero1/2 -> Subsystem1/Action
  In1/1 -> Subsystem1/1(In1), Unit Delay3/1, Do average zero1/1
  Subsystem1/1(Out1) -> Out2/1
  Do average zero1/1 -> DUMMY7/1

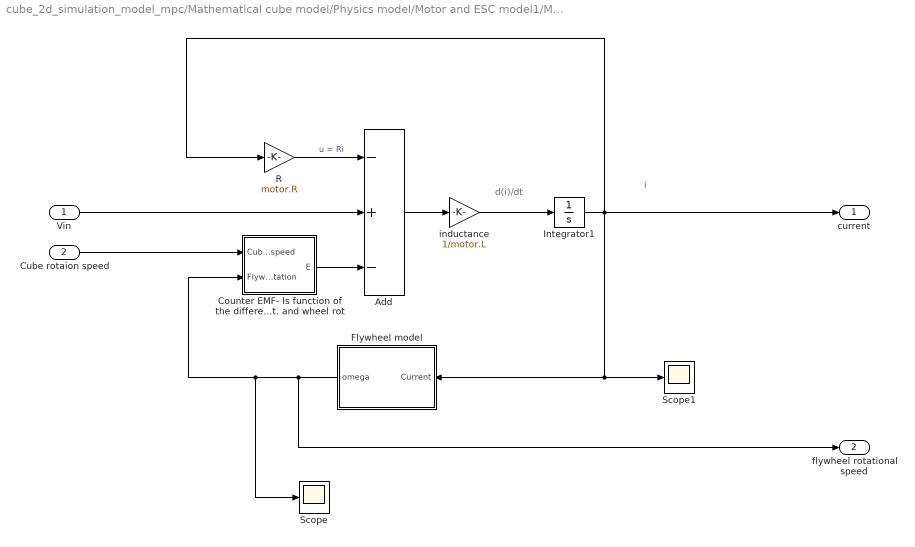
== system cube_2d_simulation_model_mpc/Mathematical cube model/Physics model/Motor and ESC model1/Motor model ==
  note: d(i)/dt
  note: i
  Vin : Inport
  Cube rotaion speed : Inport  Port=2
  Add : Sum  Inputs=-+-
  Counter EMF- Is function of the difference of the cube rot. and wheel rot : Subsystem
  Flywheel model : Subsystem
  Integrator1 : Integrator
  R : Gain  Gain=motor.R
  Scope : Scope
  Scope1 : Scope
  inductance : Gain  Gain=1/motor.L
  current : Outport
  flywheel rotational speed : Outport  Port=2
  wires:
  Counter EMF- Is function of the difference of the cube rot. and wheel rot/1(E) -> Add/3
  Flywheel model/1(omega) -> Counter EMF- Is function of the difference of the cube rot. and wheel rot/2(Flywheel rotation), Scope/1, flywheel rotational speed/1
  Cube rotaion speed/1 -> Counter EMF- Is function of the difference of the cube rot. and wheel rot/1(Cube rot speed)
  Vin/1 -> Add/2
  Integrator1/1 -> R/1, Flywheel model/1(Current), Scope1/1, current/1
  R/1 -> Add/1  "u = Ri"
  Add/1 -> inductance/1
  inductance/1 -> Integrator1/1

== system cube_2d_simulation_model_mpc/On Board Computer/PID Motor 3 DONE /Subsystem/Subsystem2 ==
  In1 : Inport
  Action Port : ActionPort  ActionType=else
  Subsystem : Subsystem
  Unit Delay1 : UnitDelay  SampleTime=-1
  Out1 : Outport
  wires:
  In1/1 -> Subsystem/1(In1)
  Subsystem/1(Average Speed) -> Out1/1  "Speed, PA1"
  Subsystem/2(One old Speed) -> Unit Delay1/1
  Unit Delay1/1 -> Subsystem/2(One old speed)

== system cube_2d_simulation_model_mpc/On Board Computer/PID Motor 3 DONE /Subsystem2/Subsystem1 ==
  In1 : Inport
  Action Port : ActionPort  ActionType=else
  Subsystem : Subsystem
  Unit Delay1 : UnitDelay  SampleTime=-1
  Out1 : Outport
  wires:
  In1/1 -> Subsystem/1(In1)
  Subsystem/1(Average Speed) -> Out1/1  "Speed, PA1"
  Subsystem/2(One old Speed) -> Unit Delay1/1
  Unit Delay1/1 -> Subsystem/2(One old speed)

== system cube_2d_simulation_model_mpc/Mathematical cube model/Physics model/Motor and ESC model1/Motor model/Counter EMF- Is function of the difference of the cube rot. and wheel rot ==
  note: The conter EMF is a bit tricky for this system, as when the stator is not fixed but moves with the cube. Therefore the rotation of the plane
      | where the stator is attached as to  be accounted for.
      |
      | Note we directly get this from an encoder in real life, as the encoder measures the velocity between the stator and the rotor.
  Cube rot speed : Inport
  Flywheel rotation : Inport  Port=2
  Add1 : Sum  Inputs=-+
  Voltage constant : Gain  Gain=motor.kt
  E : Outport
  wires:
  Voltage constant/1 -> E/1
  Add1/1 -> Voltage constant/1
  Flywheel rotation/1 -> Add1/2
  Cube rot speed/1 -> Add1/1

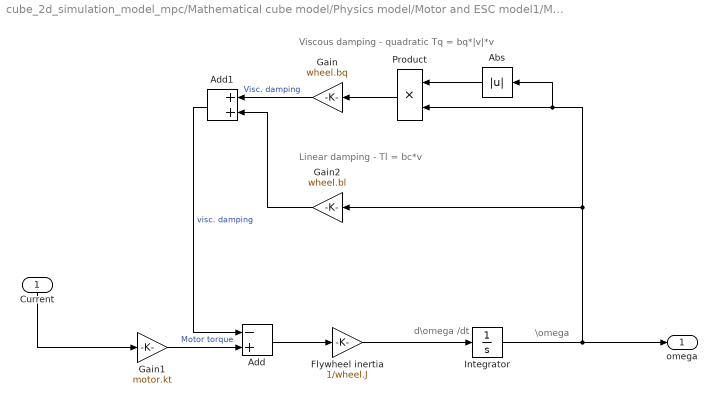
== system cube_2d_simulation_model_mpc/Mathematical cube model/Physics model/Motor and ESC model1/Motor model/Flywheel model ==
  note: Linear damping - Tl = bc*v
  note: d\omega /dt
  note: \omega
  note: Viscous damping - quadratic Tq = bq*|v|*v
  Current : Inport
  Abs : Abs
  Add : Sum  Inputs=-+
  Add1 : Sum
  Flywheel inertia : Gain  Gain=1/wheel.J
  Gain : Gain  Gain=wheel.bq
  Gain1 : Gain  Gain=motor.kt
  Gain2 : Gain  Gain=wheel.bl
  Integrator : Integrator
  Product : Product
  omega : Outport
  wires:
  Product/1 -> Gain/1
  Abs/1 -> Product/1
  Gain1/1 -> Add/2  "Motor torque"
  Add/1 -> Flywheel inertia/1
  Flywheel inertia/1 -> Integrator/1
  Current/1 -> Gain1/1
  Gain/1 -> Add1/1  "Visc. damping"
  Add1/1 -> Add/1  "visc. damping"
  Gain2/1 -> Add1/2
  Integrator/1 -> Gain2/1, Product/2, Abs/1, omega/1

== system cube_2d_simulation_model_mpc/On Board Computer/PID Motor 3 DONE /Subsystem/Subsystem2/Subsystem ==
  In1 : Inport
  One old speed : Inport  Port=2
  Add2 : Sum
  Gain2 : Gain  Gain=0.5
  Gain3 : Gain  Gain=0.5
  Average Speed : Outport
  One old Speed : Outport  Port=2
  wires:
  Add2/1 -> One old Speed/1, Average Speed/1  "Speed, PA1"
  One old speed/1 -> Gain2/1
  In1/1 -> Gain3/1
  Gain2/1 -> Add2/2
  Gain3/1 -> Add2/1

== system cube_2d_simulation_model_mpc/On Board Computer/PID Motor 3 DONE /Subsystem2/Subsystem1/Subsystem ==
  In1 : Inport
  One old speed : Inport  Port=2
  Add2 : Sum
  Gain2 : Gain  Gain=0.3
  Gain3 : Gain  Gain=0.7
  Average Speed : Outport
  One old Speed : Outport  Port=2
  wires:
  Add2/1 -> One old Speed/1, Average Speed/1  "Speed, PA1"
  One old speed/1 -> Gain2/1
  In1/1 -> Gain3/1
  Gain2/1 -> Add2/2
  Gain3/1 -> Add2/1

== matlab function cube_2d_simulation_model_mpc/On Board Computer/PID Motor 3 DONE /MATLAB Function ==
  data: activeOld input; active output; new input; old input
function active  = fcn(activeOld,new,old)
    if(new == 1 && old == 0)
        active = activeOld+0.05;
    else
        active = activeOld;
    end
end

== matlab function cube_2d_simulation_model_mpc/IMU/Transform cube states to IMU states (adds gravity) ==
  data: cube_states input Bus: CubeStates2D; imu_states output Bus: ImuStates; r_cube2imu parameter; imu_intended_alignment parameter; imu_misalignment parameter
function imu_states = CubeToImuStates(cube_states, r_cube2imu,imu_intended_alignment,imu_misalignment)
%#codegen
% Converts cube states to IMU states by changing reference frame
g = 9.82; 

persistent C_b_s; % Does not change

if isempty(C_b_s)
    C_b_s = e2t(-imu_intended_alignment-imu_misalignment); % Body to sensor. Verifiera tecken
end

% Read data
cube_angle                  = cube_states.cube_angle;
cube_angular_velocity       = cube_states.cube_angular_velocity;
cube_angular_acceleration   = cube_states.cube_angular_acceleration;

w = [0;0;cube_angular_velocity];
w_dot = [0;0;cube_angular_acceleration];
r_vec = e2t([0;0;cube_angle])*r_cube2imu;
g_vec = g*[0;1;0];

% Transformation matrices
C_i_b = e2t([0;0;-cube_angle]); % Inertial to body. Verifiera tecken

% Body reference frame, inertial coordinates
w_imu_i = [0;0;cube_angular_velocity];
a_imu_i = cross(w_dot,r_vec) + cross(w,cross(w,r_vec)) + g_vec;

% Body reference frame, sensor coordinates
w_imu_s = w_imu_i; % Rotating around the same axis
a_imu_s = C_b_s*C_i_b*a_imu_i;

% Copy to output and scale according to data sheet
imu_states.a_x = a_imu_s(1);
imu_states.a_y = a_imu_s(2);
imu_states.a_z = a_imu_s(3);

imu_states.w_x = w_imu_s(1);
imu_states.w_y = w_imu_s(2);
imu_states.w_z = w_imu_s(3);

== matlab function cube_2d_simulation_model_mpc/On Board Computer/PID Motor 3 DONE /MATLAB Function1 ==
  data: activeOld input; active output; new input; old input
function active  = fcn(activeOld,new,old)
    if(new == 1 && old == 0)
        active = activeOld-0.05;
    else
        active = activeOld;
    end
end

== matlab function cube_2d_simulation_model_mpc/Mathematical cube model/Physics model/Derivative equations ==
  data motor settings: description=Parameter struct
  data: x input; u input; x_dot output double; cube parameter; motor parameter; wheel parameter
function x_dot = CubeDerivative2D(x,u,cube, motor, wheel)
%#codegen
% x and x_dot are vectors
%% INPUTS
% - x States:
%               cube_angle
%               cube_angular_velocity
% - u           insignal, either torque or current 
% - motor       parameter struct
% - wheel       parameter struct 
% - cog_offs    simulate an offset between ideal centre of gravity and real one  


g = 9.81; 

%Using model with 2 states [theta , omega] and torque as input 
theta = x(1); 
wc    = x(2); 
 
I_2D    = cube.I_2D;            %Equivalent inertia in 2D mode
dcog    = cube.l_corner2cog;    %Distance from corner to the center of gravity of the cube center
m_tot   = cube.m_tot;           %Total cube mass
kt      = motor.kt;             %Motor torque constant 
tau_i   = motor.tau_cl;         %The motor drivers closed loop current control is approximated as a first order sytem 
J       = wheel.J;              %Wheel inertia 

%% Differential equations 
%M = kt*i;   %When current is insignal 
M = u;       %When torque is the direct insignal 

wc_dot = m_tot*dcog*g/I_2D*sin(theta)    +  M/I_2D;     %Cube 

%i_dot = i_ref/tau_i- i/tau_i;                          %Current 

x_dot = [wc; 
         wc_dot];

== matlab function cube_2d_simulation_model_mpc/Sensor simulation/Generate ideal IMU measurements ==
  data: phi input; a_out output; w input; wdot input; imu parameter; w_out output
function [a_out, w_out]  = fcn(phi, w, wdot, imu)
%#codegen

%Generate accelerometer measurements in the 2D case where the 
%cube balances on the edge and rotates around the x axis 

%Distance from corner of cube to IMU unit
d2c = imu.d2c; 

%Analytical expressions relating rotation to acceleration for this system 
ayy = -d2c*cos(phi)*w^2 - d2c*sin(phi)*wdot;
azz = d2c*cos(phi)*wdot - d2c*sin(phi)*w^2; 
 
%Add gravity 
ay = ayy + 9.81*cos(phi); 
az = azz + 9.81*sin(phi); 

%Add some noise 
a_out = [0 , [ay+0.1*randn] , [az+0.1*randn]]; 
w_out = [w+0.01*randn, 0, 0];

== matlab function cube_2d_simulation_model_mpc/Sensor simulation/Magdwick Filter ==
  data: acc input size=[1 3]; euler output; gyro input size=[1 3]; Ts_IMU input
function euler = Magdwick(acc,gyro, Ts_IMU)

    persistent AHRS;
    
    if isempty(AHRS)      
       AHRS = MadgwickAHRS('SamplePeriod', Ts_IMU, 'Beta', 0.05); 
    end
   
 
   % acc = [0 acc(2) acc(3)];   
   % gyro = [gyro(1) 0 0];       
    
    AHRS.UpdateIMU(gyro, acc);  %DEBUG
    
    q = AHRS.Quaternion;
    euler = quatern2euler(quaternConj(q));  % DEBUG -1

== matlab function cube_2d_simulation_model_mpc/Model Predictive Controller (MPC)/MPC ==
  data: cube_angle input; iref output size=1; cube_angular_velocity input; MPC parameter
function iref = MPC(cube_angle, cube_angular_velocity, MPC)

% Parameters

AA      =   single(MPC.AA);             % RHS of equality constrain before multipled with state
Linv    =   single(MPC.Linv);           % Inverse of lower-triangular Cholesky decomposition of Hessian matrix
f       =   single(MPC.f);              % Multiplier of objective function linear term
Ain     =   single(MPC.Ain);            % Linear inequality constraint coefficients
bin     =   single(MPC.bin);            % Right-hand side of inequality constraints
Aeq     =   single(MPC.Aeq);            % Linear equality constraint coefficients
iA0     =   MPC.iA0;                    % Initial active inequalities
opt     =   mpcqpsolverOptions('single');

beq  = AA*single([cube_angle;cube_angular_velocity]);   % Right-hand side of equality constraints

[z, ~, ~, ~] =  mpcqpsolver(Linv, f', Ain, bin, Aeq, beq, iA0, opt); 

iref=double(z(1));

== matlab function cube_2d_simulation_model_mpc/Mathematical cube model/Simulation control ==
  data: cube_states output; release output; x0 output; simulation_time input; cube_start_angle parameter
function [cube_states,release,x0] = SimulationControl(simulation_time,cube_start_angle)
%#codegen
% Here the initiation procedure can be programmed. 
% Current procedure: The cube lies on one side for a number of seconds
% to let the navigation algorithm find errors. Then it is placed close to
% the balancing angle and released.

deg_ = pi/180;
s_ = 1;

% type, start_time, start_angle
% time: starting time of the current pose
% angle: angle of cube
% release: if 1, the cube is allowed to move according to the physics
%          if 0, it is controlled by this procedure
% Procedure gives velocity continuous transfer between angles
% Last procedure angle gives release
procedure = [
    0*s_,   -45*deg_
    2.5*s_, -45*deg_
    3.5*s_, 45*deg_
    6*s_,   45*deg_
    7*s_,   cube_start_angle
    ];

% Read data
% Find current procedure row. Use temporary variable r_temp to convince 
% Simulink compiler that r is scalar.
r_temp = find(procedure(:,1) <= simulation_time,1,'last');
if isempty(r_temp)
    r = 1;
    disp('Warning: no valid procedure.')
else
    r = r_temp(1); % To ensure scalarity
end

if r == size(procedure,1) % last row
    release = 1;
    cube_angle = procedure(r,2);
    cube_angular_velocity = 0;
else
    release = 0;
    start_angle = procedure(r,2);
    stop_angle  = procedure(r+1,2);
    start_time  = procedure(r,1);
    stop_time   = procedure(r+1,1);

    cube_angular_velocity = (stop_angle-start_angle)/(stop_time-start_time);

    cube_angle = start_angle+(simulation_time-start_time)*cube_angular_velocity;
end

% Write data
%cube_states = [cube_angle;cube_angular_velocity;0;0;0];

cube_states = zeros(8,1);  %DEBUG!! 

if release
    %x0 = [procedure(r,2);0;0];
    x0 = [procedure(r,2);0;0;0];
else
    %x0 = zeros(3,1);
    x0 = zeros(4,1); 
end

== matlab function cube_2d_simulation_model_mpc/On Board Computer/Interface IN/MATLAB Function ==
  data: simulation_time input; y output
function y = Calibration(simulation_time)
%#codegen

if simulation_time == 0
    y = 1;
elseif simulation_time > 0 && simulation_time < 0.1
    y = 0;
elseif simulation_time > 3.5 && simulation_time < 3.7
    y = 0;
else
    y = 1;
end

== matlab function cube_2d_simulation_model_mpc/On Board Computer/MATLAB Function1 ==
  data: activeOld input; active output; new input; old input
function active  = fcn(activeOld,new,old)
    if(new == 1 && old == 0)
        if(activeOld ==0)
            active = 1;
        else 
            active = 0;
        end 
    else
        active = activeOld;
    end
end
